simulink subsystem "Chain_Drive"  (R2025b)
settings: Solver=VariableStepAuto  StartTime=0.0  StopTime=10.0  RelTol=1e-3
undefined symbols (not defined in the file): ChainFrntSprktRadius, ChainRearSprktRadius, InitRearCntctPtchLongVel, InitRearSprktAngVel, TireRearWhlInert, TireRearWhlRadius
libraries: autolibshared x1
settings Model: Creator=The MathWorks, Inc.  LastModifiedBy=The MathWorks, Inc.
settings HardwareCC: UseEmbeddedCoderFeatures=off
settings RTWCC: GPUComputeCapability=3.5

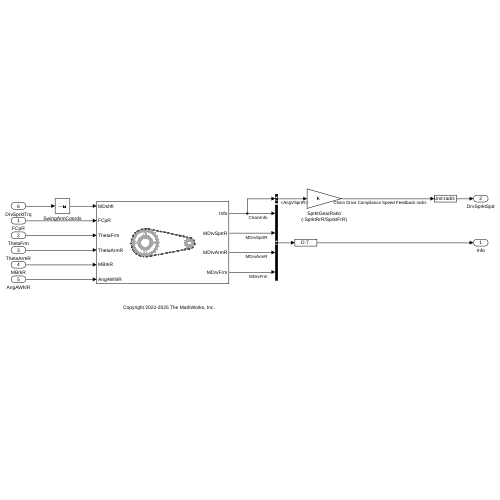
[thumbnail: Simulink's stored preview of the top-level diagram]
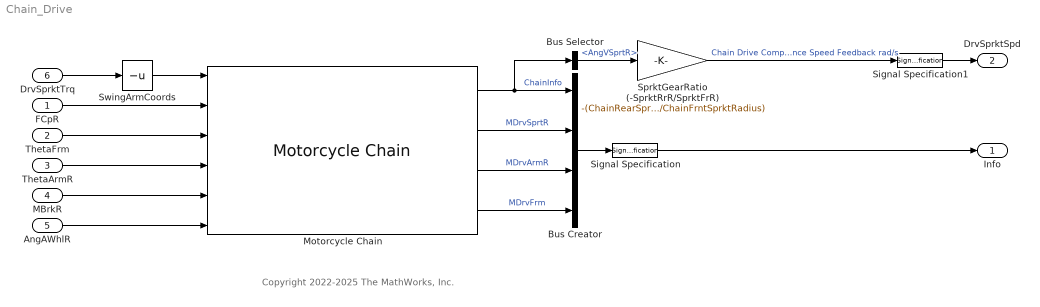
== system Chain_Drive ==
  note: Copyright 2022-2025 The MathWorks, Inc.
  FCpR : Inport
  ThetaFrm : Inport  Port=2
  ThetaArmR : Inport  Port=3
  MBrkR : Inport  Port=4
  AngAWhlR : Inport  Port=5
  DrvSprktTrq : Inport  Port=6
  Bus Creator : BusCreator  Inputs=4
  Bus Selector : BusSelector  OutputSignals=AngVSprtR
  Motorcycle Chain : autolibshared/Motorcycle Chain  aMode=2  SprktFrPxz=ChainFrntSprktCrdnt  SprktFrIyy=ChainFrntSprktInert  SprktFrR=ChainFrntSprktRadius  SprktRrIyy=ChainRearSprktInert  SprktRrR=ChainRearSprktRadius  WhlRrIyy=TireRearWhlInert(2)  WhlRrR=TireRearWhlRadius  ArmRrLen=MotoRearArmLngth  WhlDmpK=ChainWhlDamperStf  WhlDmpC=ChainWhlDamperDamp  WhlDmpAng0=ChainWhlDamperEqlbrmAng  SprktRrAngV0=InitRearSprktAngVel-InitRearCntctPtchLongVel/TireRearWhlRadius*ChainRearSprktRadius/ChainFrntSprktRadius  WhlRrAngV0=-InitRearCntctPtchLongVel/TireRearWhlRadius
      settings: LibrarySourceBlock=vdynlib/Powertrain/Drivetrain/Couplings/Motorcycle Chain
  Signal Specification : SignalSpecification  Dimensions=7
  Signal Specification1 : SignalSpecification  Unit=rad/s
  SprktGearRatio (-SprktRrR/SprktFrR) : Gain  Gain=-(ChainRearSprktRadius/ChainFrntSprktRadius)
  SwingArmCoords : UnaryMinus
  Info : Outport
  DrvSprktSpd : Outport  Port=2
  wires:
  Motorcycle Chain/1 -> Bus Creator/1, Bus Selector/1  "ChainInfo"
  FCpR/1 -> Motorcycle Chain/2
  ThetaFrm/1 -> Motorcycle Chain/3
  ThetaArmR/1 -> Motorcycle Chain/4
  MBrkR/1 -> Motorcycle Chain/5
  Signal Specification/1 -> Info/1
  Motorcycle Chain/4 -> Bus Creator/4  "MDrvFrm"
  Motorcycle Chain/3 -> Bus Creator/3  "MDrvArmR"
  Motorcycle Chain/2 -> Bus Creator/2  "MDrvSprtR"
  Bus Creator/1 -> Signal Specification/1
  Bus Selector/1 -> SprktGearRatio (-SprktRrR/SprktFrR)/1  "<AngVSprtR>"
  DrvSprktTrq/1 -> SwingArmCoords/1
  AngAWhlR/1 -> Motorcycle Chain/6
  SprktGearRatio (-SprktRrR/SprktFrR)/1 -> Signal Specification1/1  "Chain Drive Compliance Speed Feedback rad/s"
  Signal Specification1/1 -> DrvSprktSpd/1
  SwingArmCoords/1 -> Motorcycle Chain/1
